simulink model "Problem7"  (R2020b)
settings: Solver=VariableStepAuto  StartTime=0.0  StopTime=10.0  MaxStep=0.8  RelTol=1e-3
settings Model: Creator=HP  LastModifiedBy=HP

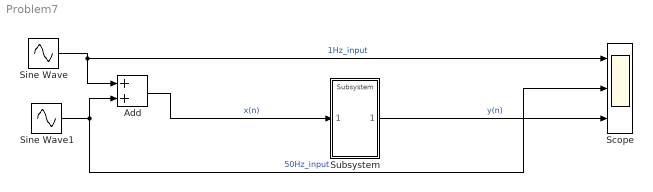
== system Problem7 ==
  Add : Sum
  Scope : Scope  NumInputPorts=3
  Sine Wave : Sin  SampleTime=0
  Sine Wave1 : Sin  Frequency=50  SampleTime=0
  Subsystem : ModelReference  ModelNameDialog=Subsystem  SimulationMode=Normal  ModelReferenceVersion=1.2
  wires:
  Sine Wave/1 -> Scope/1, Add/1  "1Hz_input"
  Sine Wave1/1 -> Add/2, Scope/2  "50Hz_input"
  Add/1 -> Subsystem/1  "x(n)"
  Subsystem/1 -> Scope/3  "y(n)"
